simulink model "simulink_builtin_sine"  (R2018b)
settings: Solver=VariableStepAuto  StartTime=0.0  StopTime=0.002  MaxStep=1e-5  MinStep=1e-4  RelTol=1e-3
libraries: commanapbnd3 x3, dspsrcs4 x1
settings Model: Creator=lenovo  LastModifiedBy=lenovo

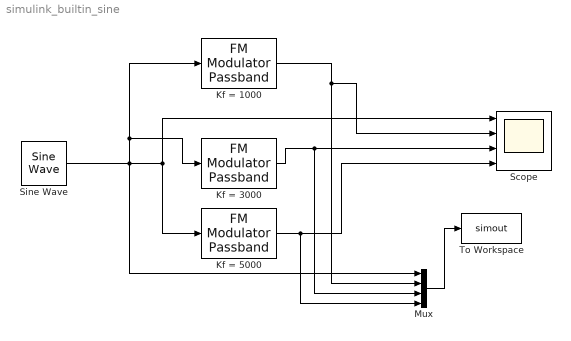
== system simulink_builtin_sine ==
  Kf = 1000 : commanapbnd3/FM Modulator Passband  Fc=10e3  Ph=0  Kc=1000
      settings: SourceProductName=Communications System Toolbox  SourceProductBaseCode=CM
  Kf = 3000 : commanapbnd3/FM Modulator Passband  Fc=10e3  Ph=0  Kc=3000
      settings: SourceProductName=Communications System Toolbox  SourceProductBaseCode=CM
  Kf = 5000 : commanapbnd3/FM Modulator Passband  Fc=10e3  Ph=0  Kc=5000
      settings: SourceProductName=Communications System Toolbox  SourceProductBaseCode=CM
  Mux : Mux
  Scope : Scope  NumInputPorts=4
  Sine Wave : dspsrcs4/Sine Wave  Amplitude=1.5  Frequency=1000  Phase=0  SampleMode=Discrete  OutComplex=Real  CompMethod=Trigonometric fcn  TableSize=Speed  SampleTime=1/1000000  SamplesPerFrame=1  ResetState=Restart at time zero  OutputFrames=off  dataType=double  wordLen=16  udDataType=sfix(16)  fracBitsMode=Best precision  numFracBits=15  OutDataTypeStr=double  LastOutDataTypeStr=double
  To Workspace : ToWorkspace  VariableName=simout  SaveFormat=Timeseries  SampleTime=-1
  wires:
  Sine Wave/1 -> Kf = 1000/1, Kf = 3000/1, Mux/1, Scope/1, Kf = 5000/1
  Kf = 1000/1 -> Mux/2, Scope/2
  Kf = 3000/1 -> Mux/3, Scope/3
  Mux/1 -> To Workspace/1
  Kf = 5000/1 -> Mux/4, Scope/4
